simulink model "segundo_controlador_sim"  (R2015a)
settings: Solver=ode45  StartTime=0.0  StopTime=80  RelTol=1e-3
libraries: cstblocks x2
settings Model: Creator=Jose Roldan  LastModifiedBy=Jose Roldan

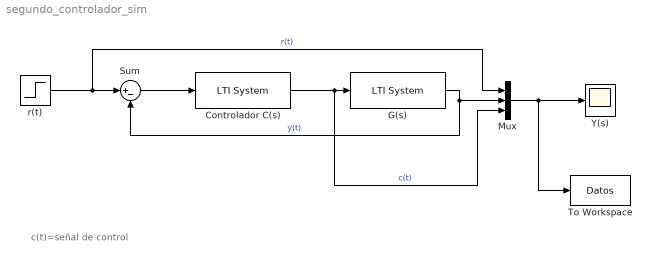
== system segundo_controlador_sim ==
  note: c(t)=señal de control
  Controlador C(s) : cstblocks/LTI System  sys=C  IC=[]
  G(s) : cstblocks/LTI System  sys=G  IC=[]
  Mux : Mux  Inputs=3
  Sum : Sum  Inputs=|+-
  To Workspace : ToWorkspace  VariableName=Datos  SaveFormat=Structure With Time  SampleTime=-1
  Y(s) : Scope
  r(t) : Step  SampleTime=0
  wires:
  Sum/1 -> Controlador C(s)/1
  Controlador C(s)/1 -> Mux/3, G(s)/1  "c(t)"
  G(s)/1 -> Sum/2, Mux/2  "y(t)"
  r(t)/1 -> Mux/1, Sum/1  "r(t)"
  Mux/1 -> To Workspace/1, Y(s)/1
